simulink model "wheel_speed"  (R2020a)
settings: Solver=ode45  StartTime=0.0  StopTime=25  MaxStep=0.1  RelTol=1e-3  AbsTol=1e-6
PostLoadFcn:
  | g = 32.18;
  | v0 = 88;
  | Rr = 15/12;  % Wheel radius
  | Kf = 1;
  | m = 50;
  | PBmax = 1500;
  | TB = 0.01;
  | I = 5;
settings Model: Creator=Jake  LastModifiedBy=Jake
settings DataIOCC: SaveOutput=off  SaveTime=off

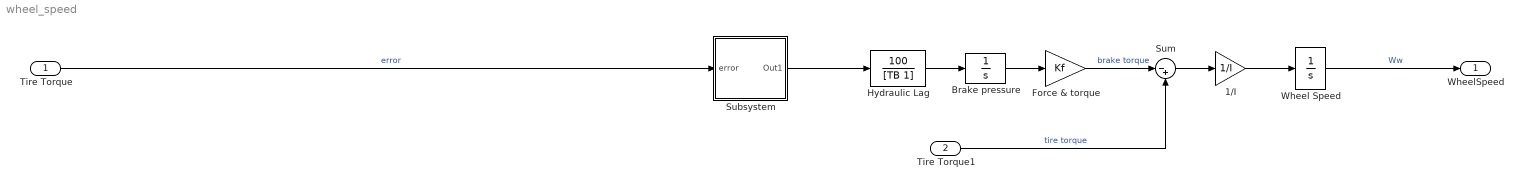
== system wheel_speed ==
  Tire Torque : Inport  OutDataTypeStr=double  PortDimensions=1  SampleTime=0
  Tire Torque1 : Inport  Port=2  OutDataTypeStr=double  PortDimensions=1  SampleTime=0
  1/I : Gain  Gain=1/I  SaturateOnIntegerOverflow=on  OutDataTypeStr=Inherit: Same as input  ParamDataTypeStr=Inherit: Same as input
  Brake pressure : Integrator  LimitOutput=on  UpperSaturationLimit=PBmax  LowerSaturationLimit=0
  Force & torque : Gain  Gain=Kf  SaturateOnIntegerOverflow=on  OutDataTypeStr=Inherit: Same as input  ParamDataTypeStr=Inherit: Same as input
  "Hydraulic Lag " : TransferFcn  Numerator=[100]  Denominator=[TB 1]
  Subsystem : Subsystem
  Sum : Sum  Inputs=|-+  InputSameDT=on  SaturateOnIntegerOverflow=on  OutDataTypeStr=Inherit: Same as first input
  Wheel Speed : Integrator  InitialCondition=v0/Rr  LimitOutput=on  UpperSaturationLimit=1000  LowerSaturationLimit=0
  WheelSpeed : Outport  OutDataTypeStr=double  PortDimensions=1  SampleTime=0  VectorParamsAs1DForOutWhenUnconnected=off
  wires:
  Tire Torque/1 -> Subsystem/1(error)  "error"
  Wheel Speed/1 -> WheelSpeed/1  "Ww"
  Sum/1 -> 1/I/1
  Brake pressure/1 -> Force & torque/1
  Force & torque/1 -> Sum/1  "brake torque"
  "Hydraulic Lag "/1 -> Brake pressure/1
  Subsystem/1(Out1) -> "Hydraulic Lag "/1
  Tire Torque1/1 -> Sum/2  "tire torque"
  1/I/1 -> Wheel Speed/1

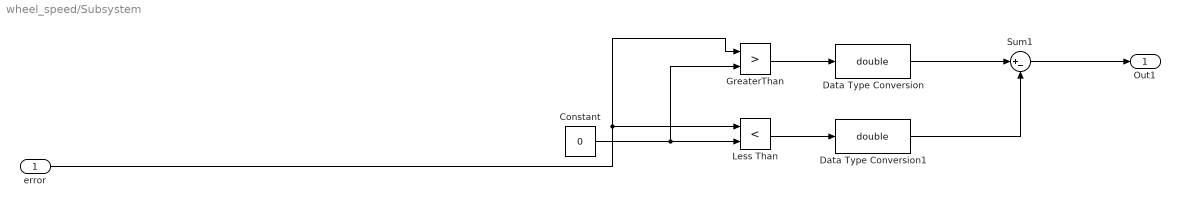
== system wheel_speed/Subsystem ==
  error : Inport  SampleTime=0
  Constant : Constant  Value=0
  Data Type Conversion : DataTypeConversion  OutDataTypeStr=double  RndMeth=Zero
  Data Type Conversion1 : DataTypeConversion  OutDataTypeStr=double  RndMeth=Zero
  GreaterThan : RelationalOperator  Operator=>  OutDataTypeStr=boolean  RndMeth=Simplest
  Less Than : RelationalOperator  Operator=<  OutDataTypeStr=boolean  RndMeth=Simplest
  Sum1 : Sum  Inputs=|+-
  Out1 : Outport
  wires:
  Data Type Conversion1/1 -> Sum1/2
  Constant/1 -> Less Than/2, GreaterThan/2
  error/1 -> Less Than/1, GreaterThan/1
  Data Type Conversion/1 -> Sum1/1
  GreaterThan/1 -> Data Type Conversion/1
  Less Than/1 -> Data Type Conversion1/1
  Sum1/1 -> Out1/1
